simulink model "DEV1ThermalModel"  (R2023b)
settings: Solver=FixedStepDiscrete  StartTime=0.0  StopTime=120  RelTol=1e-3
settings Model: Creator=schro  LastModifiedBy=mjmag
settings DataIOCC: ExternalInput=test_temp.getElement('Temp 1'),test_temp.getElement('Temp 2')  LoadExternalInput=on
settings OptimizationCC: DefaultParameterBehavior=Inlined  EnhancedBackFolding=on  PassReuseOutputArgsAs=Individual arguments  ZeroExternalMemoryAtStartup=off  ZeroInternalMemoryAtStartup=off  OptimizeBlockOrder=speed  DifferentSizesBufferReuse=on  OptimizationCustomize=off  EfficientTunableParamExpr=on
settings DebuggingCC: SolverPrmCheckMsg=warning  ParameterTunabilityLossMsg=error  StateNameClashWarn=warning
settings HardwareCC: ProdBitPerInt=16  ProdBitPerPointer=16  ProdBitPerSizeT=16  ProdBitPerPtrDiffT=16  ProdLargestAtomicFloat=None  ProdWordSize=16  ProdHWDeviceType=STMicroelectronics->ST10/Super10
settings SFSimCC: MATLABDynamicMemAlloc=off  SimTargetLang=C++
settings RTWCC: Description=Embedded Coder  SystemTargetFile=ert.tlc  TemplateMakefile=ert_default_tmf  BuildConfiguration=Faster Runs  PortableWordSizes=on  DataTypeReplacement=CDataTypesFixedWidth  TargetLang=C++
settings CodeAppCC: ForceParamTrailComments=on  IgnoreCustomStorageClasses=off  OperatorAnnotations=on  SimulinkDataObjDesc=on  SFDataObjDesc=on  MATLABFcnDesc=on  InsertBlockDesc=on  StateflowObjectComments=on  InlinedPrmAccess=Macros
settings ERTTargetCC: TargetLangStandard=C++11 (ISO)  GenerateSampleERTMain=on  CodeInterfacePackaging=C++ class  PurelyIntegerCode=on  SupportNonFinite=off  SupportComplex=off  CastingMode=Standards  ArrayLayout=Row-major  InlinedParameterPlacement=NonHierarchical  RootIOFormat=Structure reference  ERTCustomFileTemplate=example_file_process.tlc  ERTFilePackagingFormat=Compact  SuppressUnreachableDefaultCases=off  IndentSize=4  MaxIdInt64=INT64_MAX  MinIdInt64=INT64_MIN  MaxIdUint64=UINT64_MAX  MaxIdInt32=INT32_MAX  MinIdInt32=INT32_MIN  MaxIdUint32=UINT32_MAX  MaxIdInt16=INT16_MAX  MinIdInt16=INT16_MIN  MaxIdUint16=UINT16_MAX  MaxIdInt8=INT8_MAX  MinIdInt8=INT8_MIN  MaxIdUint8=UINT8_MAX

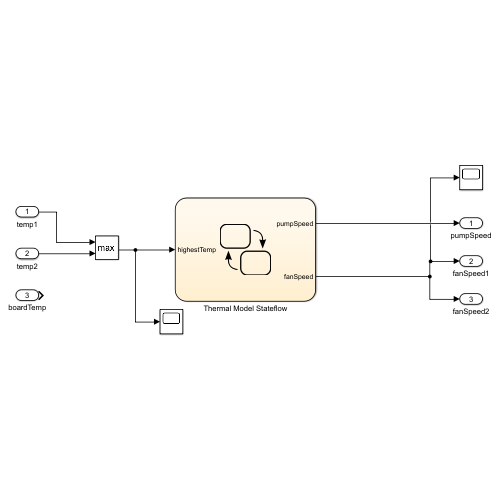
[thumbnail: Simulink's stored preview of the top-level diagram]
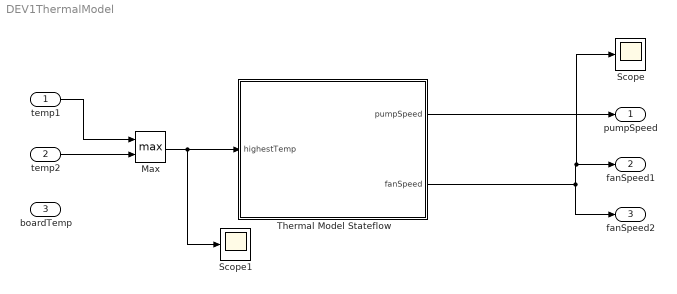
== system DEV1ThermalModel ==
  temp1 : Inport  OutDataTypeStr=uint16
  temp2 : Inport  Port=2  OutDataTypeStr=uint16
  boardTemp : Inport  Port=3  OutDataTypeStr=uint16
  Max : MinMax  Function=max  Inputs=2
  Scope : Scope
  Scope1 : Scope
  Thermal Model Stateflow : Stateflow chart  TreatAsAtomicUnit=on
  pumpSpeed : Outport  OutDataTypeStr=uint8
  fanSpeed1 : Outport  Port=2
  fanSpeed2 : Outport  Port=3
  wires:
  Thermal Model Stateflow/2(fanSpeed) -> Scope/1, fanSpeed1/1, fanSpeed2/1
  Thermal Model Stateflow/1(pumpSpeed) -> pumpSpeed/1
  Max/1 -> Scope1/1, Thermal Model Stateflow/1(highestTemp)
  temp1/1 -> Max/1
  temp2/1 -> Max/2

== stateflow chart DEV1ThermalModel/Thermal Model Stateflow ==
  state COOL_LEVEL_MAX
    pumpSpeed = 100;
    fanSpeed = 100;
  state COOL_LEVEL_1
    pumpSpeed = 75;
    fanSpeed = 75;
  state COOL_LEVEL_2
    pumpSpeed = 50;
    fanSpeed = 50;
  state COOL_LEVEL_IDLE
    pumpSpeed = 50;
    fanSpeed = 0;
  COOL_LEVEL_MAX -> COOL_LEVEL_1 : [highestTemp < 4500]
  COOL_LEVEL_1 -> COOL_LEVEL_MAX [order 1] : [highestTemp > 5000]
  COOL_LEVEL_1 -> COOL_LEVEL_2 [order 2] : [highestTemp < 3500]
  COOL_LEVEL_2 -> COOL_LEVEL_1 [order 1] : [highestTemp > 4000]
  COOL_LEVEL_2 -> COOL_LEVEL_IDLE [order 2] : [highestTemp < 2500]
  COOL_LEVEL_IDLE -> COOL_LEVEL_2 : [highestTemp > 3000]
  (default) -> COOL_LEVEL_IDLE
  data: pumpSpeed output uint8; fanSpeed output uint8; highestTemp input uint16
